simulink model "for_static_characteristic"  (R2023a)
settings: Solver=VariableStepAuto  StartTime=0.0  StopTime=10.0  RelTol=1e-3
values from neighbouring files (symbols this model uses):
  Ts = 0.1    [main.m]
settings Model: Creator=Gasper  LastModifiedBy=Gasper

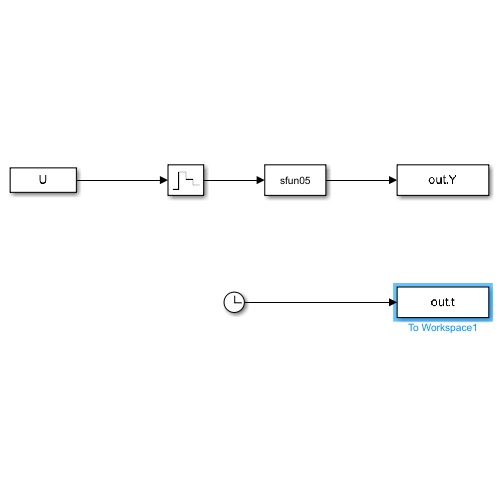
[thumbnail: Simulink's stored preview of the top-level diagram]
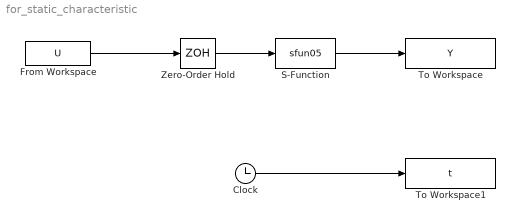
== system for_static_characteristic ==
  Clock : Clock
  From Workspace : FromWorkspace  VariableName=U  SampleTime=Ts
  S-Function : S-Function  FunctionName=sfun05  SFunctionDeploymentMode=off  EnableBusSupport=off
  To Workspace : ToWorkspace  VariableName=Y  SaveFormat=Timeseries  SampleTime=Ts
  To Workspace1 : ToWorkspace  VariableName=t  SaveFormat=Timeseries  SampleTime=Ts
  Zero-Order Hold : ZeroOrderHold  SampleTime=Ts
  wires:
  Zero-Order Hold/1 -> S-Function/1
  S-Function/1 -> To Workspace/1
  From Workspace/1 -> Zero-Order Hold/1
  Clock/1 -> To Workspace1/1
